simulink model "UseStructArrayInSF"  (R2018b)
settings: Solver=VariableStepAuto  StartTime=0.0  StopTime=10.0  RelTol=1e-3
settings Model: Creator=mganesan  LastModifiedBy=mganesan

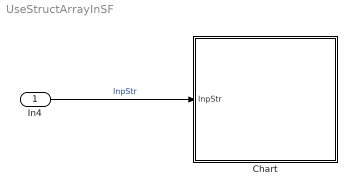
== system UseStructArrayInSF ==
  In4 : Inport  OutDataTypeStr=Bus: TempBus  BusOutputAsStruct=on
  Chart : Stateflow chart  TreatAsAtomicUnit=on
  wires:
  In4/1 -> Chart/1(InpStr)  "InpStr"

== stateflow chart UseStructArrayInSF/Chart ==
  state InitState
    en:
    x=StructArrAccess(InpStr,1);
  (default) -> InitState
  InitState -> InitState : [x.Element1==0]
  data: StrArrInp function_input type(InpStr) size=5; StrRet function_output type(InpStr); Index function_input uint32; x local type(InpStr) size=1; InpStr input
  function StrRet=StructArrAccess(StrArrInp, Index):
    | function StrRet=StructArrAccess(StrArrInp, Index)
    | StrRet = StrArrInp(Index);
    | end
